simulink model "pops"  (Simulink 6.0)
settings: Solver=ode45  SolverMode=SingleTasking  StartTime=0.0  StopTime=299  RelTol=1e-3  AbsTol=1e-6
PreLoadFcn:
  | initial_pop=20;
settings Model: Creator=The MathWorks Inc.  LastModifiedBy=batserve  ExtModeTrigMode=oneshot  ExtModeArmWhenConnect=off  ExtModeAutoUpdateStatusClock=off
settings DataIOCC: ExternalInput=[]  InitialState=[]  LimitDataPoints=off  SaveOutput=off  SaveTime=off
settings OptimizationCC: BooleanDataType=off
settings DebuggingCC: CheckExecutionContextPreStartOutputMsg=on  CheckExecutionContextRuntimeOutputMsg=on  SolverPrmCheckMsg=none  IntegerOverflowMsg=none
settings HardwareCC: TargetUnknown=on

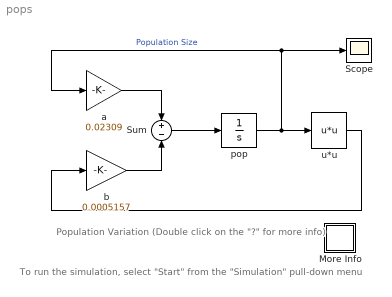
== system pops ==
  note: To run the simulation, select "Start"
      | from the "Simulation" pull-down menu
  note: Population Variation
      | (Double click on the "?" for more info)
  More Info : Subsystem  PropExecContextAcrossSSBoundary=on
      mask Display: disp('?')
  Scope : Scope
      settings: TickLabels=on  TimeRange=300  YMin=20  YMax=45  DataFormat=Array
  Sum : Sum  Inputs=+|-  SaturateOnIntegerOverflow=on  InputSameDT=on
  a : Gain  Gain=0.02309  SaturateOnIntegerOverflow=on
  b : Gain  Gain=0.0005157  SaturateOnIntegerOverflow=on
  pop : Integrator  InitialCondition=initial_pop
  u*u : Fcn  Expr=u*u
  wires:
  u*u/1 -> b/1
  a/1 -> Sum/1
  Sum/1 -> pop/1
  b/1 -> Sum/2
  pop/1 -> u*u/1, a/1, Scope/1  "Population Size"

== system pops/More Info ==
  note: This system models a population in which the number
      | of members follows the law dm/dt = a*m - b*m*m.
  note: Change the parameter initial_pop in the workspace and
      | see how the final population outcome is affected.
  note: To see a longer demo, just type "popdemo" at the command
      | line while the "pops" window is open.
